simulink model "test_controller"  (R2020a)
settings: Solver=ode1  StartTime=0.0  StopTime=100  FixedStep=0.01  RelTol=1e-3
InitFcn:
  | Initialization;
values from neighbouring files (symbols this model uses):
  g_I = [0 0 9.8]'    [Disturbance_rotor_payload_ini.m]    (also in Initialization.m = [0 0 g]'; parameter_verification_1drone.m = [0 0 g]')
  invJ_B1 = inv(J)    [Disturbance_rotor_payload_ini.m]    (also in Initialization.m)
  J = [2 0.3 -0.5;0.3 1 0.2;-0.5 0.2 3]*10^-2    [Disturbance_rotor_payload_ini.m]    (also in Initialization.m)
  K_0 = 5    [Initialization.m]
  k_L = 0.15    [Initialization.m]
  K_omega = 1*eye(3)    [Disturbance_rotor_payload_ini.m]    (also in Initialization.m)
  k_p = 0.10    (= 0.1)    [Initialization.m]
  K_q = 100    [Disturbance_rotor_payload_ini.m]    (also in Initialization.m)
  K_R = 1*eye(3)    [Disturbance_rotor_payload_ini.m]    (also in Initialization.m)
  k_v = 7    [Disturbance_rotor_payload_ini.m]    (also in Initialization.m = 0.24)
  kappa = 0.9    [Initialization.m]
  Kr = 0.2    [Initialization.m]    (also in parameter_verification_1drone.m)
  L = 1    [Disturbance_rotor_payload_ini.m]    (also in Initialization.m = 0.98; parameter_verification_1drone.m = 0.98)
  Lambda = 0.4    [Initialization.m]    (also in parameter_verification_1drone.m)
  Lambda_initalB01 = angle2quat(initial_Euler(3),initial_Euler(2),initial_Euler(1))    [Disturbance_rotor_payload_ini.m]    (also in Initialization.m)
  lambda_p = 0.2    [Disturbance_rotor_payload_ini.m]    (also in Initialization.m)
  lambda_q = 0.3    [Disturbance_rotor_payload_ini.m]    (also in Initialization.m)
  Lambda_T = 0.5    [Initialization.m]
  m_p = 0.5    [Disturbance_rotor_payload_ini.m]    (also in Initialization.m; parameter_verification_1drone.m)
  m_q = 1.63    [Disturbance_rotor_payload_ini.m]    (also in Initialization.m)
  n_1 = [0 1 0]'    [Disturbance_rotor_payload_ini.m]    (also in Initialization.m)
  omega_b01 = [0.1 0.3 0]'    [Disturbance_rotor_payload_ini.m]    (also in Initialization.m)
  P_1 = [5 0 -6]'    [Disturbance_rotor_payload_ini.m]    (also in Initialization.m)
  U_initial = [y_dot_initial;v_q]    [Disturbance_rotor_payload_ini.m]    (also in Initialization.m)
  W_p = [-0.4 0.8 -0.3]'    [Disturbance_rotor_payload_ini.m]    (also in Initialization.m)
  W_q = [-1 2 -0.3]'    [Disturbance_rotor_payload_ini.m]    (also in Initialization.m)
  X_initial = [0 0 0]'    [Disturbance_rotor_payload_ini.m]    (also in Initialization.m)
  y_inital = [0.02 -0.02]'    [Disturbance_rotor_payload_ini.m]    (also in Initialization.m)
libraries: sharedtransform x2, dspinverses x2, dspmtrx3 x1, sharedutil x1
(part 1 of 2)
settings Model: Creator=arthus  LastModifiedBy=hs293go
settings DataIOCC: ReturnWorkspaceOutputs=off
settings DebuggingCC: ArithmeticOperatorsInVariantConditions=warning
settings SFSimCC: SimUseLocalCustomCode=off  CustomCodeUndefinedFunction=UseInterfaceOnly
settings RTWCC: RTWUseLocalCustomCode=off
settings CodeAppCC: StateflowObjectComments=on

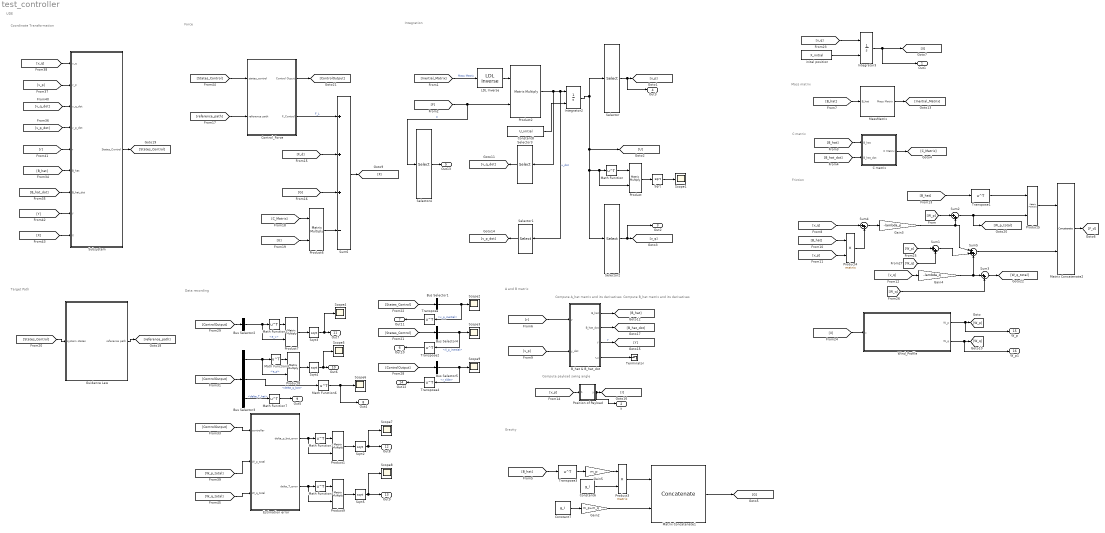
== system test_controller ==
  note: UDE
  note: Compute payload swing angle
  note: Integration
  note: Compute A_hat matrix and its derivatives
  note: Compute B_hat matrix and its derivatives
  note: Mass matrix
  note: A and B matrix
  note: Force
  note: C matrix
  note: Gravity
  note: Friction
  note: Data recording
  note: Coordinate Transformation
  note: Target Path
  B_hat & B_hat_dot : Subsystem
  Bus Selector1 : BusSelector  OutputSignals=v_p_inertial
  Bus Selector2 : BusSelector  OutputSignals=e_v
  Bus Selector3 : BusSelector  OutputSignals=e_p,delta_q_bot,delta_T_hat
  Bus Selector4 : BusSelector  OutputSignals=X_p_inertial
  Bus Selector5 : BusSelector  OutputSignals=r_tilde
  C matrix : Subsystem
  Constant6 : Constant  Value=g_I  VectorParams1D=off
  Constant7 : Constant  Value=g_I  VectorParams1D=off
  Constant8 : Constant  Value=U_initial  VectorParams1D=off
  Control_Force : Subsystem
  Estimation error : Subsystem
  Gain2 : Gain  Gain=m_p+m_q
  Gain3 : Gain  Gain=-lambda_p
  Gain4 : Gain  Gain=-lambda_q
  Gain5 : Gain  Gain=m_p
  "Guidance Law " : Subsystem
  Integrator2 : Integrator  InitialConditionSource=external  InitialCondition=U_initial
  Integrator3 : Integrator  InitialConditionSource=external
  LDL Inverse : dspinverses/LDL Inverse  errmode=Error
      settings: SourceProductBaseCode=DS
  MassMatrix : Subsystem
  Math Function{,1..4,6..7} (7 alike) : Math  Operator=transpose  SignedPower=on  SaturateOnIntegerOverflow=on
  Matrix Concatenate1 : Concatenate  Mode=Multidimensional array
  Matrix Concatenate2 : Concatenate  Mode=Multidimensional array
  Position of Payload : Subsystem
  Product{,1,3..9} (9 alike) : Product  Multiplication=Matrix(*)
  Product2 : Product  Multiplication=Matrix(*)  RndMeth=Zero
  Scope{1..9} (9 alike) : Scope
  Selector : Selector  InputPortWidth=5  IndexOptions=Index vector (dialog)  Indices=[1 2]  OutputSizes=1
  Selector1 : Selector  InputPortWidth=5  IndexOptions=Index vector (dialog)  Indices=[1 2]  OutputSizes=1
  Selector2 : Selector  InputPortWidth=5  IndexOptions=Index vector (dialog)  Indices=[3 4 5]  OutputSizes=1
  Selector3 : Selector  InputPortWidth=5  IndexOptions=Index vector (dialog)  Indices=[3 4 5]  OutputSizes=1
  Selector4 : Selector  InputPortWidth=5  IndexOptions=Index vector (dialog)  Indices=[3 4 5]  OutputSizes=1
  Sqrt{,2..5} (5 alike) : Sqrt  SaturateOnIntegerOverflow=on
  Subsystem : Subsystem
  Sum{1..4} (4 alike) : Sum  Inputs=|++
  Sum5 : Sum  Inputs=|+++
  Sum6 : Sum  Inputs=+++-
  Terminator : Terminator
  Transpose{,1..4} (5 alike) : Math  Operator=transpose  SignedPower=on  SaturateOnIntegerOverflow=on
  Wind_Profile : Subsystem
  inital position : Constant  Value=X_initial
  Out1 : Outport  SignalName=uav_pos
  y : Outport  Port=2  SignalName=pld_rel_pos
  Out2 : Outport  Port=3  SignalName=uav_vel
  Out3 : Outport  Port=4  SignalName=pld_rel_vel
  Out13 : Outport  Port=5  SignalName=act_force
  Out10 : Outport  Port=6  SignalName=pld_abs_pos
  Out11 : Outport  Port=7  SignalName=pld_abs_vel
  Out4 : Outport  Port=8  SignalName=proj_de
  Out5 : Outport  Port=9  SignalName=total_de
  Out6 : Outport  Port=10  SignalName=pos_err
  Out7 : Outport  Port=11  SignalName=vel_err
  Out8 : Outport  Port=12  SignalName=proj_de_est_err
  Out9 : Outport  Port=13  SignalName=total_de_est_err
  Out12 : Outport  Port=14  SignalName=pld_swing_est_err
  W_p : Outport  Port=15  SignalName=pld_dtb
  W_p1 : Outport  Port=16  SignalName=uav_dtb
  wires:
  ? -> ?
  Math Function7/1 -> Out5/1
  Bus Selector3/3 -> Math Function7/1  "<delta_T_hat>"
  Math Function6/1 -> Out4/1, Scope6/1
  Transpose4/1 -> Out12/1
  Bus Selector5/1 -> Transpose4/1, Scope9/1  "<r_tilde>"
  [ControlOutput] -> Bus Selector5/1
  Transpose2/1 -> Out10/1
  Transpose/1 -> Out11/1
  [W_q_total] -> Estimation error/3(W_q_total)
  Sum3/1 -> [W_q_total]
  [W_q] -> Sum3/2
  Bus Selector3/2 -> Math Function6/1  "<delta_q_bot>"
  Sqrt5/1 -> Out9/1, Scope8/1
  Estimation error/2(delta_T_error) -> Product9/2, Math Function4/1
  Math Function4/1 -> Product9/1
  Product9/1 -> Sqrt5/1
  Sqrt2/1 -> Out8/1, Scope7/1
  Estimation error/1(delta_p_bot_error) -> Product1/2, Math Function1/1
  Math Function1/1 -> Product1/1
  Product1/1 -> Sqrt2/1
  [W_p_total] -> Estimation error/2(W_p_total)
  [ControlOutput] -> Estimation error/1(controller)
  [States_Control] -> Bus Selector4/1
  Bus Selector4/1 -> Transpose2/1, Scope3/1  "<X_p_inertial>"
  Bus Selector1/1 -> Transpose/1, Scope2/1  "<v_p_inertial>"
  [States_Control] -> Bus Selector1/1
  [ControlOutput] -> Bus Selector3/1
  [ControlOutput] -> Bus Selector2/1
  Math Function3/1 -> Product8/1
  Bus Selector3/1 -> Product8/2, Math Function3/1  "<e_p>"
  Sqrt4/1 -> Out6/1, Scope5/1
  Product8/1 -> Sqrt4/1
  Bus Selector2/1 -> Product7/2, Math Function2/1  "<e_v>"
  Sqrt3/1 -> Out7/1, Scope4/1
  Product7/1 -> Sqrt3/1
  Math Function2/1 -> Product7/1
  Control_Force/1(Control Ouput) -> [ControlOutput]
  Control_Force/2(F_Control) -> Sum6/1  "F_L"
  [States_Control] -> "Guidance Law "/1(system states)
  "Guidance Law "/1(reference path) -> [reference_path]
  [reference_path] -> Control_Force/2(reference path)
  [X] -> Subsystem/9(X)
  [Y] -> Subsystem/8(Y)
  [r] -> Subsystem/5(r)
  [v_q_dot] -> Subsystem/3(v_q_dot)
  [v_q] -> Subsystem/1(v_q)
  [v_p] -> Subsystem/2(v_p)
  [v_p_dot] -> Subsystem/4(v_p_dot)
  [B_hat] -> Subsystem/6(B_hat)
  [B_hat_dot] -> Subsystem/7(B_hat_dot)
  Subsystem/1(States_Control) -> [States_Control]
  Selector1/1 -> [v_p_dot]
  Selector3/1 -> [v_q_dot]
  Selector/1 -> Out3/1, [v_p]
  [X] -> Wind_Profile/1(x)
  Wind_Profile/2(W_q) -> W_p1/1, [W_q]
  Sqrt/1 -> Scope1/1
  Product/1 -> Sqrt/1
  Math Function/1 -> Product/1
  [W_p] -> Sum1/1
  [W_q] -> Sum1/2
  [W_p] -> Sum2/1
  Wind_Profile/1(W_p) -> W_p/1, [W_p]
  B_hat & B_hat_dot/3(Y) -> [Y]  "Y"
  Gain3/1 -> Sum2/2, Sum5/1
  Sum2/1 -> [W_p_total], Product5/2
  Sum1/1 -> Sum5/2
  Gain4/1 -> Sum3/1, Sum5/3
  Integrator3/1 -> Out1/1, [X]
  B_hat & B_hat_dot/4(r_z) -> Terminator/1
  [States_Control] -> Control_Force/1(states_control)
  Constant8/1 -> Integrator2/2
  [v_q] -> Integrator3/1
  inital position/1 -> Integrator3/2
  Product6/1 -> Sum6/4
  [U] -> Product6/2
  [C_Matrix] -> Product6/1
  [G] -> Sum6/3
  [F_d] -> Sum6/2
  Sum6/1 -> [F]
  [v_p] -> Position of Payload/1(y_dot)
  Position of Payload/1(y) -> y/1, [r]
  Product5/1 -> Matrix Concatenate2/1
  Transpose1/1 -> Product5/1
  [B_hat] -> Transpose1/1
  [v_q] -> Gain4/1
  Product4/1 -> Sum4/2
  [v_p] -> Product4/2
  [B_hat] -> Product4/1
  [v_q] -> Sum4/1
  Sum4/1 -> Gain3/1
  Sum5/1 -> Matrix Concatenate2/2
  Matrix Concatenate2/1 -> [F_d]
  Matrix Concatenate1/1 -> [G]
  Gain2/1 -> Matrix Concatenate1/2
  Constant7/1 -> Gain2/1
  Product3/1 -> Matrix Concatenate1/1
  Transpose3/1 -> Gain5/1
  Constant6/1 -> Product3/2
  Gain5/1 -> Product3/1
  [B_hat] -> Transpose3/1
  [B_hat_dot] -> C matrix/2(B_hat_dot)
  [B_hat] -> C matrix/1(B_hat)
  C matrix/1(C Matrix) -> [C_Matrix]
  Selector2/1 -> Out2/1, [v_q]
  Integrator2/1 -> Selector/1, [U], Product/2, Math Function/1, Selector2/1
  Product2/1 -> Selector3/1, Selector1/1, Integrator2/1  "u_dot"
  [F] -> Selector4/1, Product2/2  "F"
  [Inertial_Matrix] -> LDL Inverse/1  "Mass Matrix"
  LDL Inverse/1 -> Product2/1
  [B_hat] -> MassMatrix/1(B_hat)
  [v_p] -> B_hat & B_hat_dot/2(y_dot)
  [r] -> B_hat & B_hat_dot/1(y)
  B_hat & B_hat_dot/1(B_hat) -> [B_hat]
  B_hat & B_hat_dot/2(B_hat_dot) -> [B_hat_dot]
  MassMatrix/1(Mass Matrix) -> [Inertial_Matrix]
  Selector4/1 -> Out13/1

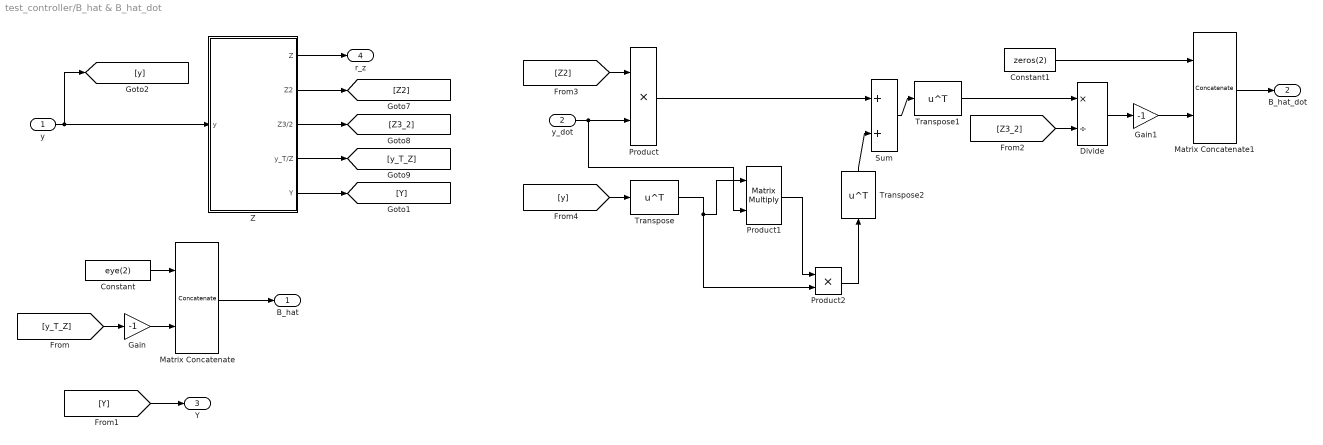
== system test_controller/B_hat & B_hat_dot ==
  y : Inport
  y_dot : Inport  Port=2
  Constant : Constant  Value=eye(2)
  Constant1 : Constant  Value=zeros(2)
  Divide : Product  Inputs=*/
  Gain : Gain  Gain=-1
  Gain1 : Gain  Gain=-1
  Matrix Concatenate : Concatenate  Mode=Multidimensional array
  Matrix Concatenate1 : Concatenate  Mode=Multidimensional array
  Product : Product  RndMeth=Zero
  Product1 : Product  Multiplication=Matrix(*)  RndMeth=Zero
  Product2 : Product  RndMeth=Zero
  Sum : Sum
  Transpose : Math  Operator=transpose  SignedPower=on  SaturateOnIntegerOverflow=on
  Transpose1 : Math  Operator=transpose  SignedPower=on  SaturateOnIntegerOverflow=on
  Transpose2 : Math  Operator=transpose  SignedPower=on  SaturateOnIntegerOverflow=on
  Z : Subsystem
  B_hat : Outport  VectorParamsAs1DForOutWhenUnconnected=off
  B_hat_dot : Outport  Port=2  VectorParamsAs1DForOutWhenUnconnected=off
  Y : Outport  Port=3  VectorParamsAs1DForOutWhenUnconnected=off
  r_z : Outport  Port=4  VectorParamsAs1DForOutWhenUnconnected=off
  wires:
  y_dot/1 -> Product/2, Product1/2
  y/1 -> Z/1(y), [y]
  Matrix Concatenate/1 -> B_hat/1
  Matrix Concatenate1/1 -> B_hat_dot/1
  Z/1(Z) -> r_z/1
  Z/2(Z2) -> [Z2]
  Z/3(Z3/2) -> [Z3_2]
  Z/4(y_T/Z) -> [y_T_Z]
  [y_T_Z] -> Gain/1
  Constant/1 -> Matrix Concatenate/1
  Gain/1 -> Matrix Concatenate/2
  Z/5(Y) -> [Y]
  [Y] -> Y/1
  Constant1/1 -> Matrix Concatenate1/1
  [Z3_2] -> Divide/2
  Sum/1 -> Transpose1/1
  [Z2] -> Product/1
  [y] -> Transpose/1
  Transpose/1 -> Product1/1, Product2/2
  Product1/1 -> Product2/1
  Divide/1 -> Gain1/1
  Gain1/1 -> Matrix Concatenate1/2
  Product2/1 -> Transpose2/1
  Product/1 -> Sum/1
  Transpose1/1 -> Divide/1
  Transpose2/1 -> Sum/2

== system test_controller/C matrix ==
  B_hat : Inport
  B_hat_dot : Inport  Port=2
  Constant : Constant  Value=[zeros(2,3);zeros(3)]  VectorParams1D=off
  Gain4 : Gain  Gain=m_p
  Gain5 : Gain  Gain=m_p
  Matrix Concatenate : Concatenate  Mode=Multidimensional array  ConcatenateDimension=2
  Matrix Concatenate1 : Concatenate  Mode=Multidimensional array
  Product1 : Product  Multiplication=Matrix(*)
  Transpose3 : Math  Operator=transpose  SignedPower=on  SaturateOnIntegerOverflow=on
  C Matrix : Outport  VectorParamsAs1DForOutWhenUnconnected=off
  wires:
  Matrix Concatenate/1 -> C Matrix/1
  Matrix Concatenate1/1 -> Matrix Concatenate/1
  Constant/1 -> Matrix Concatenate/2
  B_hat/1 -> Transpose3/1
  Transpose3/1 -> [B_hatT]
  Gain5/1 -> Matrix Concatenate1/1
  [B_hatT] -> Product1/1
  B_hat_dot/1 -> Gain4/1, Product1/2
  Product1/1 -> Gain5/1
  Gain4/1 -> Matrix Concatenate1/2

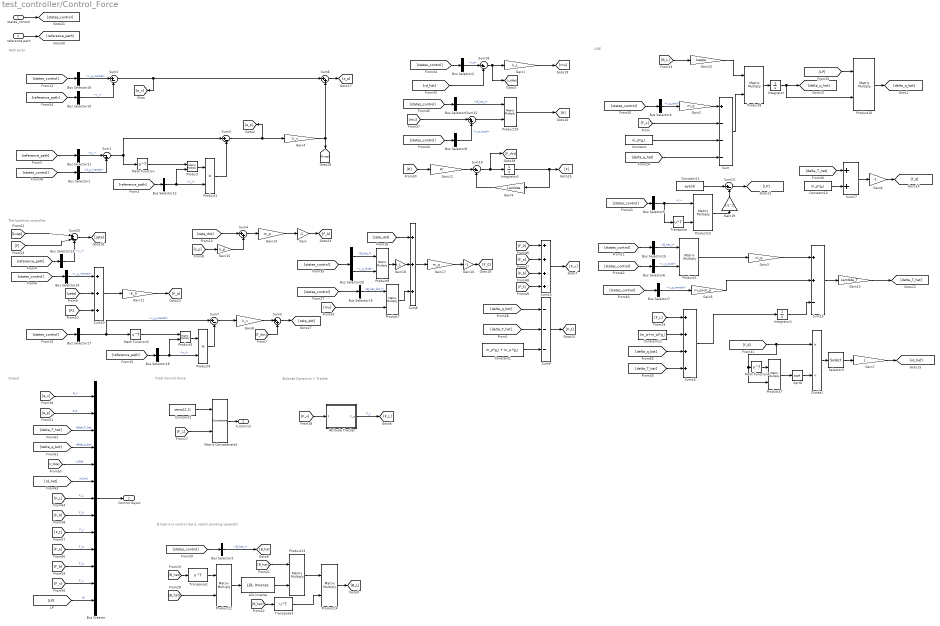
== system test_controller/Control_Force ==
  note: Output
  note: Path error
  note: The baseline controller
  note: Attitude Dynamics + Tracker
  note: B matrix in control law (L vector pointing upwards)
  note: UDE
  note: Total Control Force
  states_control : Inport
  reference path : Inport  Port=2
  Attitude Tracker : Subsystem
  Bus Creator : BusCreator  Inputs=13
  Bus Selector1 : BusSelector  OutputSignals=X_p_inertial
  Bus Selector10 : BusSelector  OutputSignals=v_i
  Bus Selector11 : BusSelector  OutputSignals=p_i
  Bus Selector12 : BusSelector  OutputSignals=n_i
  Bus Selector13 : BusSelector  OutputSignals=v_i
  Bus Selector{7,14,16..17} (4 alike) : BusSelector  OutputSignals=v_p_inertial
  Bus Selector15 : BusSelector  OutputSignals=B_hat_l
  Bus Selector18 : BusSelector  OutputSignals=n_i
  Bus Selector19 : BusSelector  OutputSignals=B_hat_dot_l
  Bus Selector2 : BusSelector  OutputSignals=r_q
  Bus Selector20 : BusSelector  OutputSignals=B_hat_l,v_q_local
  Bus Selector3 : BusSelector  OutputSignals=B_hat_l
  Bus Selector4 : BusSelector  OutputSignals=v_q_dot
  Bus Selector5 : BusSelector  OutputSignals=L
  Bus Selector6 : BusSelector  OutputSignals=v_q_local
  Bus Selector8 : BusSelector  OutputSignals=v_q_local
  Bus Selector9 : BusSelector  OutputSignals=B_hat_l
  Constant : Constant  Value=m_q*g_I
  Constant1 : Constant  Value=m_p*g_I + m_q *g_I
  Constant11 : Constant  Value=eye(3)
  Constant12 : Constant  Value=(m_p+m_q)*g_I
  Constant13 : Constant  Value=m_p*g_I
  Constant2 : Constant  Value=zeros(2,1)
  Divide1 : Product  Inputs=*/
  Gain : Gain  Gain=-1
  Gain1 : Gain  Gain=k_L
  Gain10 : Gain  Gain=kappa
  Gain11 : Gain  Gain=-K_0
  Gain12 : Gain  Gain=Kr
  Gain13 : Gain  Gain=Lambda_T
  Gain14 : Gain  Gain=m_p
  Gain15 : Gain  Gain=k_p
  Gain16 : Gain  Gain=-1
  Gain17 : Gain  Gain=m_q
  Gain18 : Gain  Gain=k_L
  Gain19 : Gain  Gain=1/L^2
  Gain2 : Gain  Gain=m_q
  Gain3 : Gain  Gain=m_q
  Gain4 : Gain  Gain=k_v
  Gain5 : Gain  Gain=m_q+m_p
  Gain6 : Gain  Gain=-1
  Gain7 : Gain  Gain=L
  Gain8 : Gain  Gain=k_v
  Gain9 : Gain  Gain=Lambda
  Integrator : Integrator
  Integrator1 : Integrator
  Integrator2 : Integrator
  LDL Inverse : dspinverses/LDL Inverse  errmode=Error
      settings: SourceProductBaseCode=DS
  Math Function : Math  Operator=transpose  SignedPower=on  SaturateOnIntegerOverflow=on
  Math Function3 : Math  Operator=transpose  SignedPower=on  SaturateOnIntegerOverflow=on
  Math Function4 : Math  Operator=transpose  SignedPower=on  SaturateOnIntegerOverflow=on
  Matrix Concatenate1 : Concatenate  Mode=Multidimensional array
  Product{,2..3,7..9,12..17,19} (13 alike) : Product  Multiplication=Matrix(*)
  Product1 : Product
  Product4 : Product
  Selector3 : Selector  InputPortWidth=3  IndexOptions=Index vector (dialog)  Indices=[1 2]  OutputSizes=1
  Sqrt6 : Sqrt  SaturateOnIntegerOverflow=on
  Sum : Sum  Inputs=+---
  Sum1 : Sum  Inputs=|-+
  Sum10 : Sum  Inputs=+++
  Sum{4..6,12} (4 alike) : Sum  Inputs=|++
  Sum{2..3,7,13,18..19} (6 alike) : Sum  Inputs=|+-
  Sum14 : Sum  Inputs=++++
  Sum15 : Sum  Inputs=++-
  Sum16 : Sum  Inputs=++++
  Sum17 : Sum
  Sum20 : Sum  Inputs=|++-
  Sum8 : Sum  Inputs=+++
  Sum9 : Sum  Inputs=---
  Transpose : Math  Operator=transpose  SignedPower=on  SaturateOnIntegerOverflow=on
  Transpose1 : Math  Operator=transpose  SignedPower=on  SaturateOnIntegerOverflow=on
  Transpose3 : Math  Operator=transpose  SignedPower=on  SaturateOnIntegerOverflow=on
  Control Ouput : Outport  VectorParamsAs1DForOutWhenUnconnected=off
  F_Control : Outport  Port=2  VectorParamsAs1DForOutWhenUnconnected=off
  wires:
  Constant2/1 -> Matrix Concatenate1/1
  Sum3/1 -> [e_p], Gain4/1
  Sum1/1 -> Sum3/1, Math Function/1
  Math Function/1 -> Product/1
  Product/1 -> Product1/1
  Product1/1 -> Sum3/2
  Bus Selector6/1 -> Product2/2  "<v_q_local>"
  Bus Selector7/1 -> Gain5/1  "<v_p_inertial>"
  Matrix Concatenate1/1 -> F_Control/1
  Attitude Tracker/1(F_q) -> [F_L]  "F_L"
  Sum2/1 -> [e_v], Sum6/1
  [F_L] -> Matrix Concatenate1/2
  [F_v] -> Attitude Tracker/1(F)
  Sum14/1 -> [F_v]
  [B_hat] -> Transpose1/1
  Transpose1/1 -> Product12/1
  [B_hat] -> Product12/2
  Product12/1 -> LDL Inverse/1
  LDL Inverse/1 -> Product13/2
  [B_hat] -> Product13/1
  Transpose3/1 -> Product14/2
  [B_hat] -> Transpose3/1
  Product13/1 -> Product14/1
  Product14/1 -> [B_L]
  [B_L] -> Gain10/1
  Gain10/1 -> Product8/1
  Integrator/1 -> Product16/2, [delta_q_hat]
  [delta_q_hat] -> Sum/4
  Constant/1 -> Sum/3
  [F_L] -> Sum/2
  Gain2/1 -> Sum/1
  Sum/1 -> Product8/2
  Product8/1 -> Integrator/1
  Constant11/1 -> Sum13/1
  Product15/1 -> Gain19/1
  Sum13/1 -> [LP]
  [LP] -> Product16/1
  Product16/1 -> [delta_q_bot]
  Bus Selector15/1 -> Product2/1  "<B_hat_l>"
  Product2/1 -> Gain3/1
  Gain3/1 -> Sum15/1
  Gain5/1 -> Sum15/2
  Sum15/1 -> Gain13/1
  Integrator1/1 -> Sum15/3
  [F_L] -> Sum16/1
  Constant12/1 -> Sum16/2
  [delta_q_bot] -> Sum16/3
  [delta_T_hat] -> Sum16/4
  [delta_T_hat] -> Sum17/1
  Constant13/1 -> Sum17/2
  Sum17/1 -> Gain6/1
  Gain6/1 -> [f_d]
  Selector3/1 -> Gain7/1
  Gain7/1 -> [rd_hat]
  Product17/1 -> Sqrt6/1
  [f_d] -> Product17/2, Math Function4/1, Divide1/1
  Divide1/1 -> Selector3/1
  Sqrt6/1 -> Divide1/2
  Math Function4/1 -> Product17/1
  Sum6/1 -> [s_p]
  Bus Selector16/1 -> Sum2/1  "<v_p_inertial>"
  Sum18/1 -> [r_tilde], Gain1/1
  Gain1/1 -> [mu]
  states_control/1 -> [states_control]
  [states_control] -> Bus Selector1/1
  Bus Selector1/1 -> Sum1/2  "<X_p_inertial>"
  [states_control] -> Bus Selector2/1
  Bus Selector2/1 -> Sum18/1  "<r_q>"
  [states_control] -> Bus Selector3/1
  Bus Selector3/1 -> [B_hat]  "<B_hat_l>"
  [states_control] -> Bus Selector4/1
  Bus Selector4/1 -> Gain2/1  "<v_q_dot>"
  [states_control] -> Bus Selector5/1
  Bus Selector5/1 -> Product15/1, Transpose/1  "<L>"
  [states_control] -> Bus Selector6/1
  [states_control] -> Bus Selector7/1
  [mu] -> Sum12/1
  Bus Selector8/1 -> Sum12/2  "<v_q_local>"
  [states_control] -> Bus Selector8/1
  Sum12/1 -> Product19/2
  Bus Selector9/1 -> Product19/1  "<B_hat_l>"
  [states_control] -> Bus Selector9/1
  Product19/1 -> [R]
  [F_0] -> Sum14/1
  [F_a] -> Sum14/2
  [F_b] -> Sum14/3
  [F_t] -> Sum14/4
  Integrator2/1 -> Gain9/1, [F]
  Sum19/1 -> [F_dot], Integrator2/1
  Gain9/1 -> Sum19/2
  [R] -> Gain12/1
  Gain12/1 -> Sum19/1
  Sum20/1 -> [zeta]
  Gain4/1 -> [kvep], Sum6/2
  [kvep] -> Sum20/1
  [F] -> Sum20/2
  reference path/1 -> [reference_path]
  [reference_path] -> Bus Selector10/1
  Bus Selector10/1 -> Sum2/2  "<v_i>"
  Bus Selector11/1 -> Sum1/1  "<p_i>"
  [reference_path] -> Bus Selector11/1
  [reference_path] -> Bus Selector12/1
  Bus Selector12/1 -> Product/2, Product1/2  "<n_i>"
  [reference_path] -> Bus Selector13/1
  Bus Selector13/1 -> Sum20/3  "<v_i>"
  Sum4/1 -> Gain14/1
  Gain16/1 -> [F_0]
  Gain11/1 -> [F_a]
  Sum9/1 -> [F_t]
  Sum10/1 -> Gain11/1
  Constant1/1 -> Sum9/3
  [states_control] -> Bus Selector14/1
  Bus Selector14/1 -> Sum10/1  "<v_p_inertial>"
  [zeta] -> Sum10/2
  [R] -> Sum10/3
  Sum16/1 -> Integrator1/1
  [delta_q_bot] -> Sum9/1
  [rd_hat] -> Sum18/2
  Gain13/1 -> [delta_T_hat]
  [states_control] -> Bus Selector15/1
  [delta_T_hat] -> Sum9/2
  [states_control] -> Bus Selector16/1
  Gain/1 -> [F_b]
  [F_dot] -> Sum5/2
  Sum5/1 -> [zeta_dot]
  [zeta_dot] -> Sum4/1
  Gain14/1 -> Gain/1
  Gain15/1 -> Sum4/2
  [s_p] -> Gain15/1
  Gain8/1 -> Sum5/1
  [states_control] -> Bus Selector17/1
  Bus Selector17/1 -> Sum7/1, Math Function3/1  "<v_p_inertial>"
  [reference_path] -> Bus Selector18/1
  Bus Selector18/1 -> Product3/2, Product4/2  "<n_i>"
  Product3/1 -> Product4/1
  Math Function3/1 -> Product3/1
  Product4/1 -> Sum7/2
  Sum7/1 -> Gain8/1
  Gain17/1 -> Gain16/1
  Sum8/1 -> Gain17/1
  [zeta_dot] -> Sum8/1
  Gain18/1 -> Sum8/2
  [states_control] -> Bus Selector19/1
  Bus Selector19/1 -> Product7/1  "<B_hat_dot_l>"
  Product7/1 -> Sum8/3
  [mu] -> Product7/2
  Product9/1 -> Gain18/1
  Bus Selector20/1 -> Product9/1  "<B_hat_l>"
  [states_control] -> Bus Selector20/1
  Bus Selector20/2 -> Product9/2  "<v_q_local>"
  Bus Creator/1 -> Control Ouput/1
  [e_v] -> Bus Creator/1  "e_v"
  [e_p] -> Bus Creator/2  "e_p"
  [delta_T_hat] -> Bus Creator/3  "delta_T_hat"
  [delta_q_bot] -> Bus Creator/4  "delta_q_bot"
  [r_tilde] -> Bus Creator/5  "r_tilde"
  [rd_hat] -> Bus Creator/6  "rd_hat"
  [F_L] -> Bus Creator/7  "F_L"
  [F_0] -> Bus Creator/8  "F_0"
  [F_t] -> Bus Creator/9  "F_t"
  [F_a] -> Bus Creator/10  "F_a"
  [F_b] -> Bus Creator/11  "F_b"
  [F_v] -> Bus Creator/12  "F_v"
  [LP] -> Bus Creator/13  "LP"
  Gain19/1 -> Sum13/2
  Transpose/1 -> Product15/2

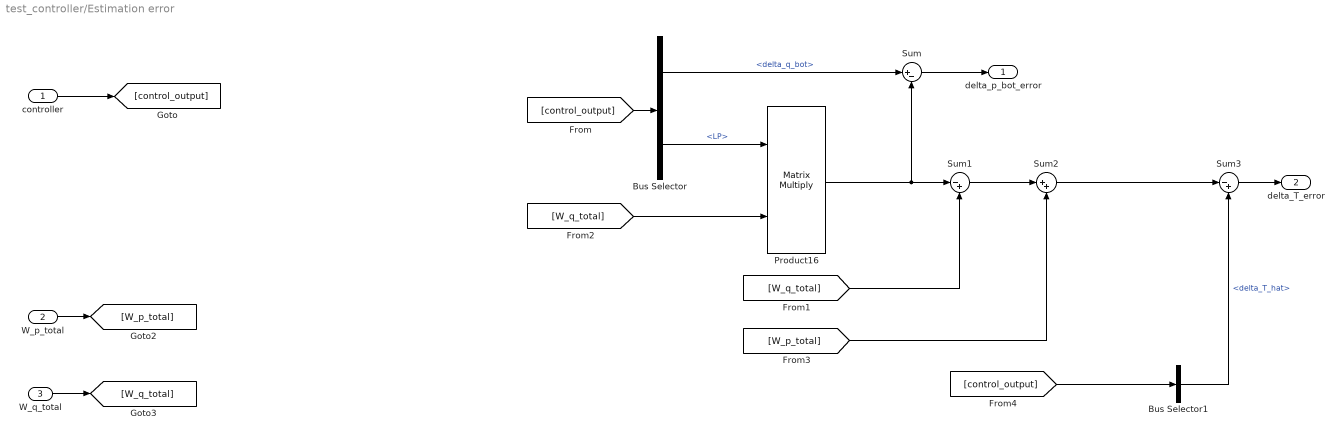
== system test_controller/Estimation error ==
  controller : Inport
  W_p_total : Inport  Port=2
  W_q_total : Inport  Port=3
  Bus Selector : BusSelector  OutputSignals=delta_q_bot,LP
  Bus Selector1 : BusSelector  OutputSignals=delta_T_hat
  Product16 : Product  Multiplication=Matrix(*)
  Sum : Sum  Inputs=|+-
  Sum1 : Sum  Inputs=|-+
  Sum2 : Sum  Inputs=|++
  Sum3 : Sum  Inputs=|-+
  delta_p_bot_error : Outport  VectorParamsAs1DForOutWhenUnconnected=off
  delta_T_error : Outport  Port=2  VectorParamsAs1DForOutWhenUnconnected=off
  wires:
  controller/1 -> [control_output]
  W_p_total/1 -> [W_p_total]
  W_q_total/1 -> [W_q_total]
  [control_output] -> Bus Selector/1
  Bus Selector/1 -> Sum/1  "<delta_q_bot>"
  Bus Selector/2 -> Product16/1  "<LP>"
  [W_q_total] -> Product16/2
  Product16/1 -> Sum1/1, Sum/2
  Sum/1 -> delta_p_bot_error/1
  Sum3/1 -> delta_T_error/1
  [W_q_total] -> Sum1/2
  Sum1/1 -> Sum2/1
  [W_p_total] -> Sum2/2
  Sum2/1 -> Sum3/1
  [control_output] -> Bus Selector1/1
  Bus Selector1/1 -> Sum3/2  "<delta_T_hat>"

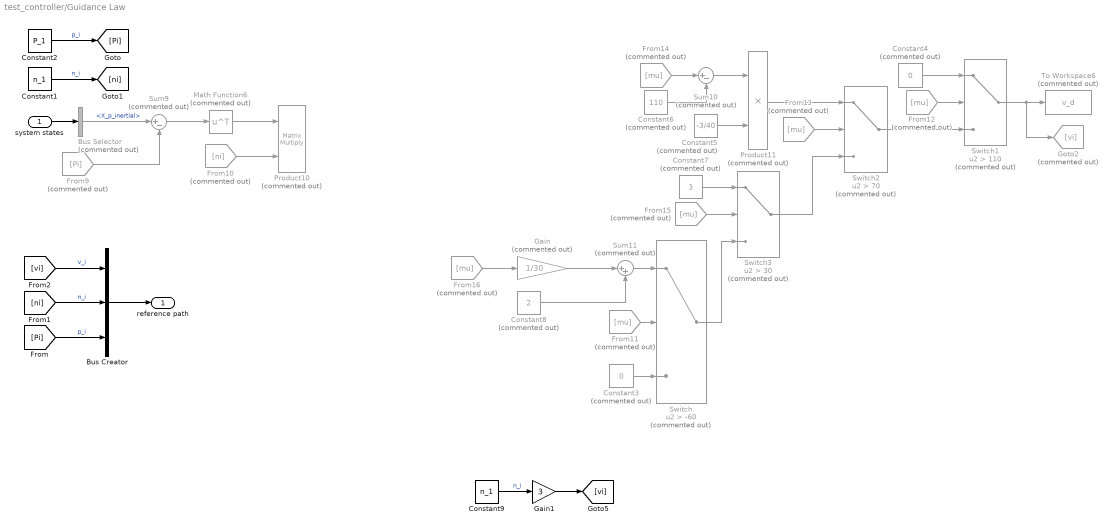
== system test_controller/Guidance Law  ==
  system states : Inport
  Bus Creator : BusCreator  Inputs=3
  Bus Selector : BusSelector  Commented=on  OutputSignals=X_p_inertial
  Constant1 : Constant  Value=n_1
  Constant2 : Constant  Value=P_1
  Constant3 : Constant  Commented=on  Value=0
  Constant4 : Constant  Commented=on  Value=0
  Constant5 : Constant  Commented=on  Value=-3/40
  Constant6 : Constant  Commented=on  Value=110
  Constant7 : Constant  Commented=on  Value=3
  Constant8 : Constant  Commented=on  Value=2
  Constant9 : Constant  Value=n_1
  From10 : From  Commented=on  GotoTag=ni
  From{11..16} (6 alike) : From  Commented=on  GotoTag=mu
  From9 : From  Commented=on  GotoTag=Pi
  Gain : Gain  Commented=on  Gain=1/30
  Gain1 : Gain  Gain=3
  Goto2 : Goto  Commented=on  GotoTag=vi
  Math Function6 : Math  Commented=on  Operator=transpose  SignedPower=on  SaturateOnIntegerOverflow=on
  Product10 : Product  Commented=on  Multiplication=Matrix(*)
  Product11 : Product  Commented=on
  Sum10 : Sum  Commented=on  Inputs=|+-
  Sum11 : Sum  Commented=on  Inputs=|++
  Sum9 : Sum  Commented=on  Inputs=|+-
  Switch : Switch  Commented=on  Criteria=u2 > Threshold  Threshold=-60
  Switch1 : Switch  Commented=on  Criteria=u2 > Threshold  Threshold=110
  Switch2 : Switch  Commented=on  Criteria=u2 > Threshold  Threshold=70
  Switch3 : Switch  Commented=on  Criteria=u2 > Threshold  Threshold=30
  To Workspace6 : ToWorkspace  Commented=on  VariableName=v_d  SaveFormat=Structure With Time  SampleTime=-1
  reference path : Outport  VectorParamsAs1DForOutWhenUnconnected=off
  wires:
  Sum11/1 -> Switch/1
  Math Function6/1 -> Product10/1
  From10/1 -> Product10/2
  Constant8/1 -> Sum11/2
  From9/1 -> Sum9/2
  Constant7/1 -> Switch3/1
  From13/1 -> Switch2/2
  Product11/1 -> Switch2/1
  Constant5/1 -> Product11/2
  From14/1 -> Sum10/1
  Switch2/1 -> Switch1/3
  Gain/1 -> Sum11/1
  Switch3/1 -> Switch2/3
  From16/1 -> Gain/1
  Constant4/1 -> Switch1/1
  Switch/1 -> Switch3/3
  Sum10/1 -> Product11/1
  Switch1/1 -> Goto2/1, To Workspace6/1
  Sum9/1 -> Math Function6/1
  From12/1 -> Switch1/2
  Constant6/1 -> Sum10/2
  From11/1 -> Switch/2
  From15/1 -> Switch3/2
  Bus Selector/1 -> Sum9/1  "<X_p_inertial>"
  Bus Creator/1 -> reference path/1
  Constant2/1 -> [Pi]  "p_i"
  system states/1 -> Bus Selector/1
  [Pi] -> Bus Creator/3  "p_i"
  Constant1/1 -> [ni]  "n_i"
  [ni] -> Bus Creator/2  "n_i"
  [vi] -> Bus Creator/1  "v_i"
  Constant3/1 -> Switch/3
  Constant9/1 -> Gain1/1  "n_i"
  Gain1/1 -> [vi]

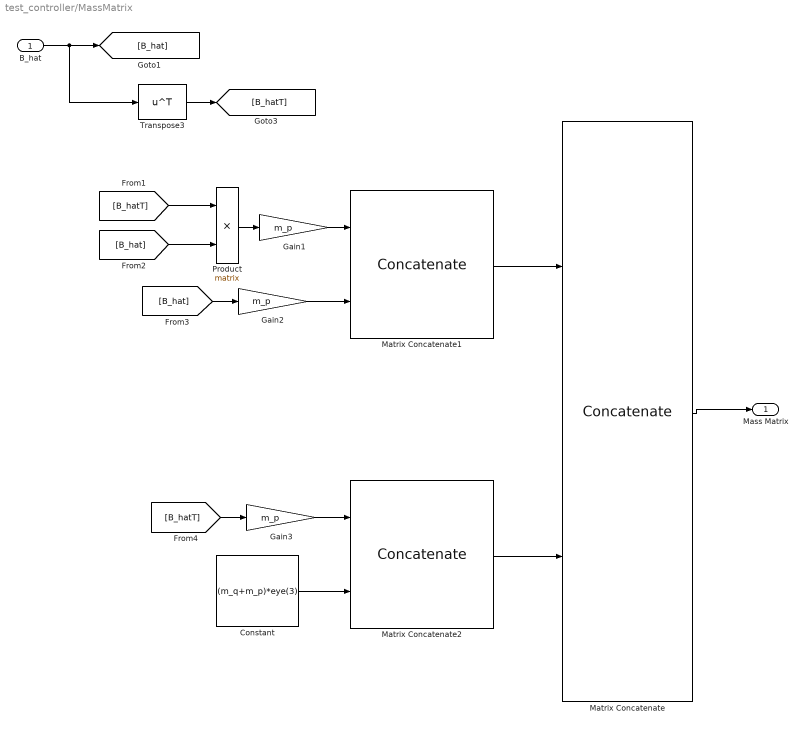
== system test_controller/MassMatrix ==
  B_hat : Inport
  Constant : Constant  Value=(m_q+m_p)*eye(3)
  Gain1 : Gain  Gain=m_p
  Gain2 : Gain  Gain=m_p
  Gain3 : Gain  Gain=m_p
  Matrix Concatenate : Concatenate  Mode=Multidimensional array  ConcatenateDimension=2
  Matrix Concatenate1 : Concatenate  Mode=Multidimensional array
  Matrix Concatenate2 : Concatenate  Mode=Multidimensional array
  Product : Product  Multiplication=Matrix(*)
  Transpose3 : Math  Operator=transpose  SignedPower=on  SaturateOnIntegerOverflow=on
  Mass Matrix : Outport  VectorParamsAs1DForOutWhenUnconnected=off
  wires:
  Matrix Concatenate/1 -> Mass Matrix/1
  Matrix Concatenate1/1 -> Matrix Concatenate/1
  Matrix Concatenate2/1 -> Matrix Concatenate/2
  B_hat/1 -> [B_hat], Transpose3/1
  Transpose3/1 -> [B_hatT]
  [B_hatT] -> Product/1
  [B_hat] -> Product/2
  Product/1 -> Gain1/1
  Gain1/1 -> Matrix Concatenate1/1
  Gain2/1 -> Matrix Concatenate1/2
  [B_hat] -> Gain2/1
  Constant/1 -> Matrix Concatenate2/2
  [B_hatT] -> Gain3/1
  Gain3/1 -> Matrix Concatenate2/1

== system test_controller/Position of Payload ==
  y_dot : Inport
  Integrator : Integrator  InitialConditionSource=external
  inital position : Constant  Value=y_inital  VectorParams1D=off
  y : Outport  VectorParamsAs1DForOutWhenUnconnected=off
  wires:
  Integrator/1 -> y/1
  y_dot/1 -> Integrator/1
  inital position/1 -> Integrator/2

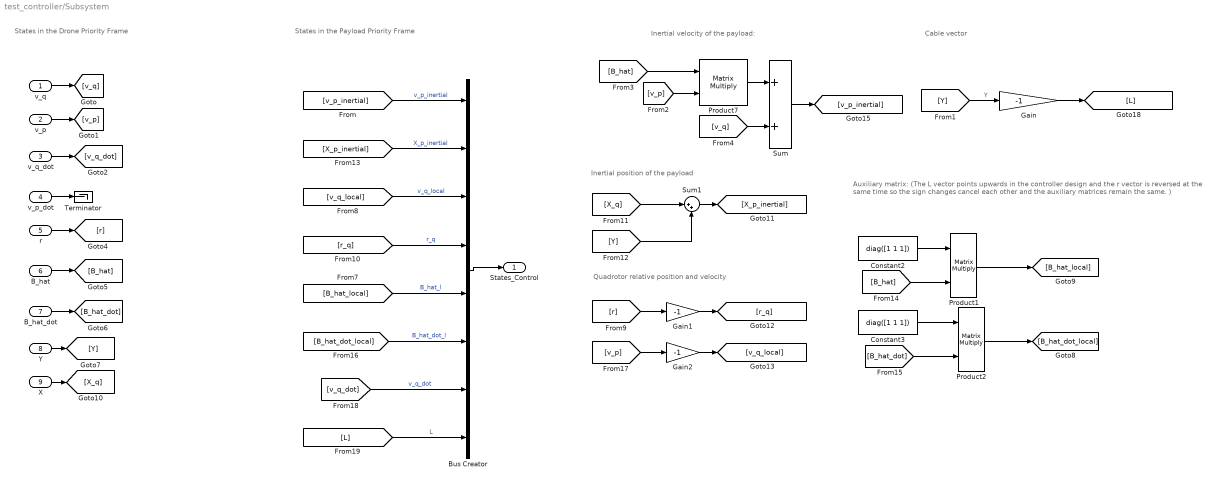
== system test_controller/Subsystem ==
  note: Quadrotor relative position and velocity
  note: Auxiliary matrix: (The L vector points upwards in the controller design and the r vector is reversed at the same time so
      | the sign changes cancel each other and the auxiliary matrices remain the same.  )
  note: Inertial position of the payload
  note: Cable vector
  note: Inertial velocity of the payload:
  note: States in the Drone Priority Frame
  note: States in the Payload Priority Frame
  v_q : Inport
  v_p : Inport  Port=2
  v_q_dot : Inport  Port=3
  v_p_dot : Inport  Port=4
  r : Inport  Port=5
  B_hat : Inport  Port=6
  B_hat_dot : Inport  Port=7
  Y : Inport  Port=8
  X : Inport  Port=9
  Bus Creator : BusCreator  Inputs=8
  Constant2 : Constant  Value=diag([1 1 1])
  Constant3 : Constant  Value=diag([1 1 1])
  Gain : Gain  Gain=-1
  Gain1 : Gain  Gain=-1
  Gain2 : Gain  Gain=-1
  Product1 : Product  Multiplication=Matrix(*)
  Product2 : Product  Multiplication=Matrix(*)
  Product7 : Product  Multiplication=Matrix(*)
  Sum : Sum
  Sum1 : Sum  Inputs=|++
  Terminator : Terminator
  States_Control : Outport  VectorParamsAs1DForOutWhenUnconnected=off
  wires:
  Bus Creator/1 -> States_Control/1
  Product7/1 -> Sum/1
  Sum/1 -> [v_p_inertial]
  [v_q] -> Sum/2
  [Y] -> Gain/1  "Y"
  Gain/1 -> [L]
  v_q/1 -> [v_q]
  v_p/1 -> [v_p]
  v_q_dot/1 -> [v_q_dot]
  v_p_dot/1 -> Terminator/1
  r/1 -> [r]
  B_hat/1 -> [B_hat]
  B_hat_dot/1 -> [B_hat_dot]
  Y/1 -> [Y]
  X/1 -> [X_q]
  [X_q] -> Sum1/1
  [Y] -> Sum1/2
  Sum1/1 -> [X_p_inertial]
  [r] -> Gain1/1
  Gain1/1 -> [r_q]
  [v_p_inertial] -> Bus Creator/1  "v_p_inertial"
  [X_p_inertial] -> Bus Creator/2  "X_p_inertial"
  [v_q_local] -> Bus Creator/3  "v_q_local"
  [r_q] -> Bus Creator/4  "r_q"
  [B_hat_local] -> Bus Creator/5  "B_hat_l"
  [B_hat_dot_local] -> Bus Creator/6  "B_hat_dot_l"
  [B_hat] -> Product1/2
  Product1/1 -> [B_hat_local]
  [B_hat_dot] -> Product2/2
  Product2/1 -> [B_hat_dot_local]
  [v_p] -> Gain2/1
  Gain2/1 -> [v_q_local]
  [v_q_dot] -> Bus Creator/7  "v_q_dot"
  [L] -> Bus Creator/8  "L"
  [v_p] -> Product7/2
  [B_hat] -> Product7/1
  Constant2/1 -> Product1/1
  Constant3/1 -> Product2/1

== system test_controller/Wind_Profile ==
  note: Constant wind profile is used
  x : Inport
  Constant1 : Constant  Value=W_p
  Constant2 : Constant  Value=W_q
  Terminator : Terminator
  W_p : Outport  VectorParamsAs1DForOutWhenUnconnected=off
  W_q : Outport  Port=2  VectorParamsAs1DForOutWhenUnconnected=off
  wires:
  x/1 -> Terminator/1
  Constant2/1 -> W_q/1
  Constant1/1 -> W_p/1

== system test_controller/B_hat & B_hat_dot/Z ==
  y : Inport
  Constant : Constant  Value=L^2  VectorParams1D=off
  Divide : Product  Inputs=*/
  Dot Product : DotProduct  InputSameDT=on  OutDataTypeStr=Inherit: Inherit via internal rule
  Dot Product1 : DotProduct  InputSameDT=on  OutDataTypeStr=Inherit: Inherit via internal rule
  Matrix Concatenate : Concatenate  ConcatenateDimension=2
  Sqrt : Sqrt  SaturateOnIntegerOverflow=on
  Sum : Sum  Inputs=|-+
  Transpose2 : Math  Operator=transpose  SignedPower=on  SaturateOnIntegerOverflow=on
  Z : Outport  VectorParamsAs1DForOutWhenUnconnected=off
  Z2 : Outport  Port=2  VectorParamsAs1DForOutWhenUnconnected=off
  Z3/2 : Outport  Port=3  VectorParamsAs1DForOutWhenUnconnected=off
  y_T/Z : Outport  Port=4  VectorParamsAs1DForOutWhenUnconnected=off
  Y : Outport  Port=5  VectorParamsAs1DForOutWhenUnconnected=off
  wires:
  y/1 -> Divide/1, Matrix Concatenate/1, Dot Product/2, Dot Product/1
  Constant/1 -> Sum/2
  Dot Product/1 -> Sum/1
  Sum/1 -> Sqrt/1, Z2/1, Dot Product1/2
  Sqrt/1 -> Dot Product1/1, Divide/2, Z/1, Matrix Concatenate/2
  Dot Product1/1 -> Z3/2/1
  Divide/1 -> Transpose2/1
  Transpose2/1 -> y_T/Z/1
  Matrix Concatenate/1 -> Y/1

== system test_controller/Control_Force/Attitude Tracker ==
  F : Inport
  Attitude Dynamics : Subsystem
  Attitude Tracker : Subsystem
  Atttitude Extraction : Subsystem
  Constant : Constant  Value=[0 0 1]'  VectorParams1D=off
  Divide : Product  Inputs=*/
  Dot Product : DotProduct  InputSameDT=on  OutDataTypeStr=Inherit: Inherit via internal rule
  Product : Product  Multiplication=Matrix(*)
  Product1 : Product
  Sqrt : Sqrt  SaturateOnIntegerOverflow=on
  Terminator : Terminator
  Terminator1 : Terminator
  F_q : Outport  VectorParamsAs1DForOutWhenUnconnected=off
  wires:
  F/1 -> Dot Product/2, Dot Product/1, Divide/1
  Constant/1 -> Product/2
  Product/1 -> Product1/2  "n_z"
  Product1/1 -> F_q/1
  Sqrt/1 -> Product1/1, Divide/2
  Dot Product/1 -> Sqrt/1
  Atttitude Extraction/1(R_d) -> Attitude Tracker/1(R_d)
  Atttitude Extraction/2(omega_d) -> Attitude Tracker/2(omega_d)
  Atttitude Extraction/3(omega_d_dot) -> Attitude Tracker/3(omega_d_dot)
  Divide/1 -> Atttitude Extraction/1(n_d)  "n1"
  Attitude Dynamics/4(omega_b) -> Attitude Tracker/5(omega)
  Attitude Dynamics/3(Euler) -> Terminator1/1  "Euler"
  Attitude Dynamics/2(RBI) -> Terminator/1
  Attitude Tracker/1(Torque_in_body_frame) -> Attitude Dynamics/1(MB)  "Mq_b"
  Attitude Dynamics/1(RIB) -> Attitude Tracker/4(R), Product/1  "IRB"

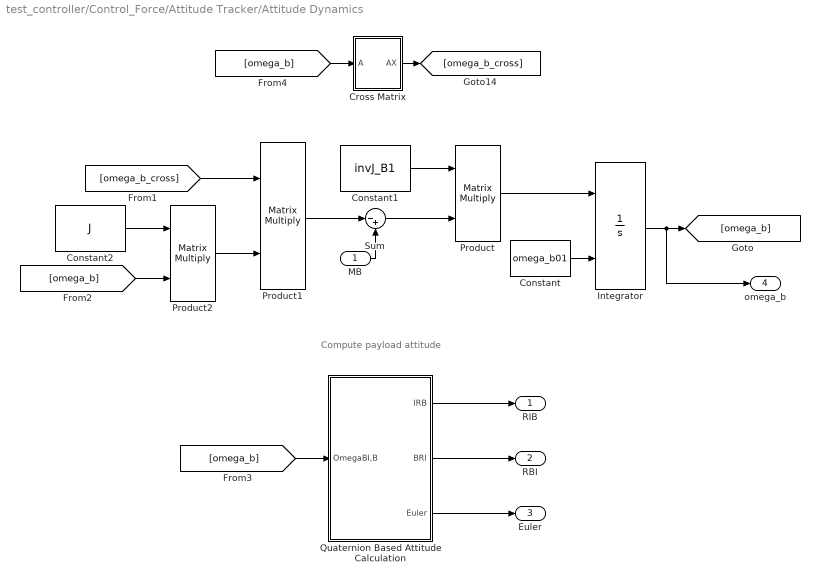
== system test_controller/Control_Force/Attitude Tracker/Attitude Dynamics ==
  note: Compute payload attitude
  MB : Inport
  Constant : Constant  Value=omega_b01  VectorParams1D=off
  Constant1 : Constant  Value=invJ_B1  VectorParams1D=off
  Constant2 : Constant  Value=J  VectorParams1D=off
  Cross Matrix : Subsystem
  Integrator : Integrator  InitialConditionSource=external
  Product : Product  Multiplication=Matrix(*)
  Product1 : Product  Multiplication=Matrix(*)
  Product2 : Product  Multiplication=Matrix(*)
  Quaternion Based Attitude Calculation : Subsystem
  Sum : Sum  Inputs=|-+
  RIB : Outport  VectorParamsAs1DForOutWhenUnconnected=off
  RBI : Outport  Port=2  VectorParamsAs1DForOutWhenUnconnected=off
  Euler : Outport  Port=3  VectorParamsAs1DForOutWhenUnconnected=off
  omega_b : Outport  Port=4  VectorParamsAs1DForOutWhenUnconnected=off
  wires:
  [omega_b] -> Cross Matrix/1(A)
  Cross Matrix/1(AX) -> [omega_b_cross]
  [omega_b] -> Quaternion Based Attitude Calculation/1(OmegaBI,B)
  Quaternion Based Attitude Calculation/1(IRB) -> RIB/1
  Quaternion Based Attitude Calculation/2(BRI) -> RBI/1
  Quaternion Based Attitude Calculation/3(Euler) -> Euler/1
  Integrator/1 -> omega_b/1, [omega_b]
  Constant/1 -> Integrator/2
  Product/1 -> Integrator/1
  Constant1/1 -> Product/1
  Sum/1 -> Product/2
  MB/1 -> Sum/2
  [omega_b_cross] -> Product1/1
  Product2/1 -> Product1/2
  Constant2/1 -> Product2/1
  [omega_b] -> Product2/2
  Product1/1 -> Sum/1

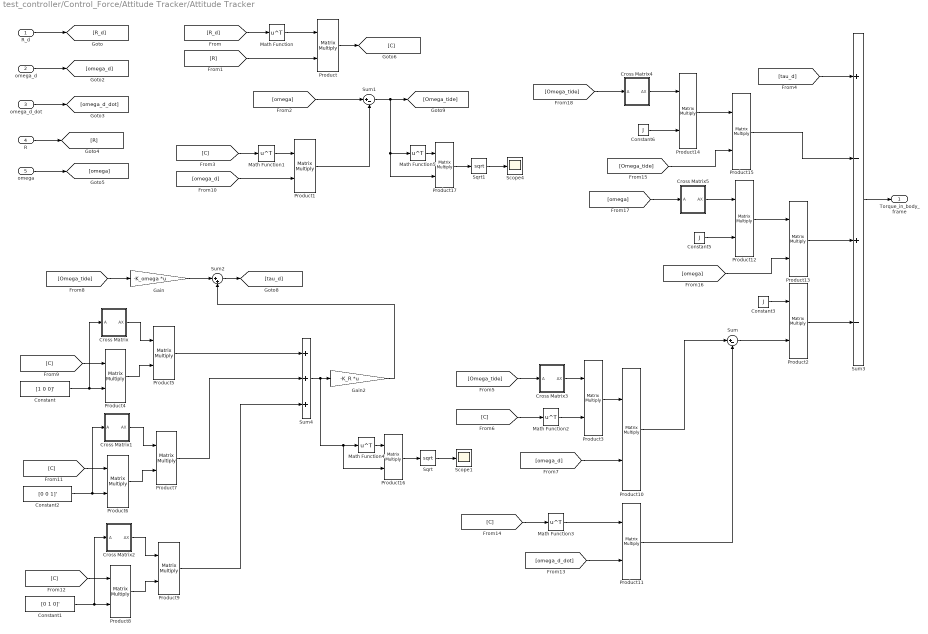
== system test_controller/Control_Force/Attitude Tracker/Attitude Tracker ==
  R_d : Inport
  omega_d : Inport  Port=2
  omega_d_dot : Inport  Port=3
  R : Inport  Port=4
  omega : Inport  Port=5
  Constant : Constant  Value=[1 0 0]'
  Constant1 : Constant  Value=[0 1 0]'
  Constant2 : Constant  Value=[0 0 1]'
  Constant3 : Constant  Value=J  VectorParams1D=off
  Constant5 : Constant  Value=J  VectorParams1D=off
  Constant6 : Constant  Value=J  VectorParams1D=off
  Cross Matrix : Subsystem
  Cross Matrix1 : Subsystem
  Cross Matrix2 : Subsystem
  Cross Matrix3 : Subsystem
  Cross Matrix4 : Subsystem
  Cross Matrix5 : Subsystem
  Gain : Gain  Gain=-K_omega  Multiplication=Matrix(K*u)
  Gain2 : Gain  Gain=-K_R  Multiplication=Matrix(K*u)
  Math Function{,1..5} (6 alike) : Math  Operator=transpose  SignedPower=on  SaturateOnIntegerOverflow=on
  Product{,1..17} (18 alike) : Product  Multiplication=Matrix(*)
  Scope1 : Scope
  Scope4 : Scope
  Sqrt : Sqrt  SaturateOnIntegerOverflow=on
  Sqrt1 : Sqrt  SaturateOnIntegerOverflow=on
  Sum : Sum  Inputs=|+-
  Sum1 : Sum  Inputs=|+-
  Sum2 : Sum  Inputs=|++
  Sum3 : Sum  Inputs=+-+-
  Sum4 : Sum  Inputs=+++
  Torque_in_body_frame : Outport  VectorParamsAs1DForOutWhenUnconnected=off
  wires:
  R_d/1 -> [R_d]
  omega_d/1 -> [omega_d]
  omega_d_dot/1 -> [omega_d_dot]
  [R_d] -> Math Function/1
  Math Function/1 -> Product/1
  R/1 -> [R]
  omega/1 -> [omega]
  [R] -> Product/2
  Product/1 -> [C]
  [C] -> Math Function1/1
  Math Function1/1 -> Product1/1
  [omega] -> Sum1/1
  Product1/1 -> Sum1/2
  [omega_d] -> Product1/2
  Sum2/1 -> [tau_d]
  Gain/1 -> Sum2/1
  [Omega_tide] -> Gain/1
  [tau_d] -> Sum3/1
  [C] -> Product4/1
  Constant/1 -> Cross Matrix/1(A), Product4/2
  Cross Matrix/1(AX) -> Product5/1
  Product4/1 -> Product5/2
  [C] -> Product6/1
  Constant2/1 -> Cross Matrix1/1(A), Product6/2
  Cross Matrix1/1(AX) -> Product7/1
  Product6/1 -> Product7/2
  Product7/1 -> Sum4/2
  [C] -> Product8/1
  Constant1/1 -> Cross Matrix2/1(A), Product8/2
  Cross Matrix2/1(AX) -> Product9/1
  Product8/1 -> Product9/2
  Product9/1 -> Sum4/3
  Product5/1 -> Sum4/1
  Gain2/1 -> Sum2/2
  Sum3/1 -> Torque_in_body_frame/1
  Constant3/1 -> Product2/1
  Sum/1 -> Product2/2
  [Omega_tide] -> Cross Matrix3/1(A)
  [C] -> Math Function2/1
  Cross Matrix3/1(AX) -> Product3/1
  Math Function2/1 -> Product3/2
  Product3/1 -> Product10/1
  [omega_d] -> Product10/2
  Product10/1 -> Sum/1
  [C] -> Math Function3/1
  Math Function3/1 -> Product11/1
  [omega_d_dot] -> Product11/2
  Product11/1 -> Sum/2
  Product2/1 -> Sum3/4
  Product13/1 -> Sum3/3
  Product12/1 -> Product13/1
  [omega] -> Product13/2
  [omega] -> Cross Matrix5/1(A)
  Cross Matrix5/1(AX) -> Product12/1
  Constant5/1 -> Product12/2
  Product14/1 -> Product15/1
  [Omega_tide] -> Product15/2
  [Omega_tide] -> Cross Matrix4/1(A)
  Cross Matrix4/1(AX) -> Product14/1
  Constant6/1 -> Product14/2
  Product15/1 -> Sum3/2
  Sum4/1 -> Product16/2, Math Function4/1, Gain2/1
  Math Function4/1 -> Product16/1
  Product16/1 -> Sqrt/1
  Sqrt/1 -> Scope1/1
  Sum1/1 -> Math Function5/1, Product17/2, [Omega_tide]
  Math Function5/1 -> Product17/1
  Product17/1 -> Sqrt1/1
  Sqrt1/1 -> Scope4/1

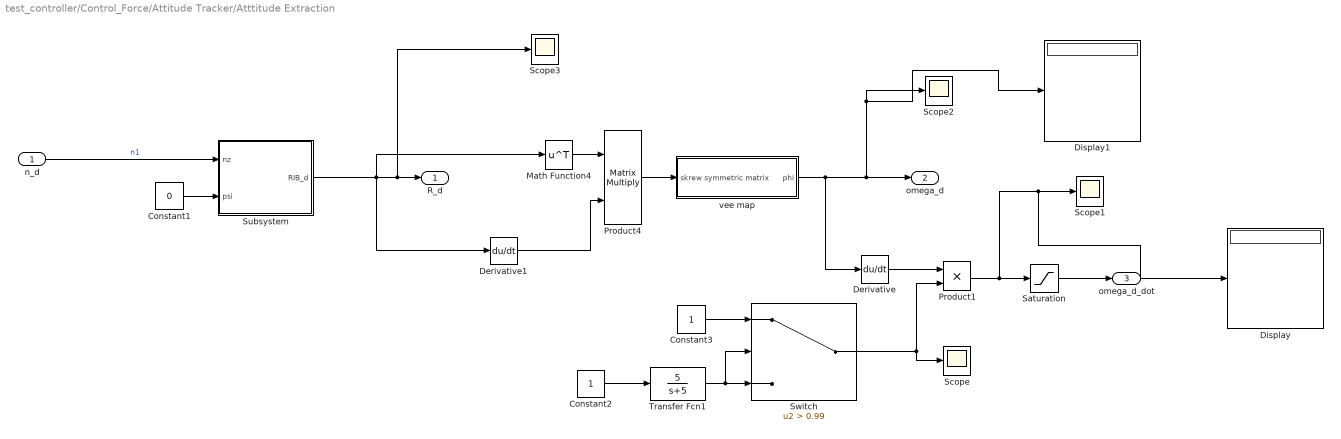
== system test_controller/Control_Force/Attitude Tracker/Atttitude Extraction ==
  n_d : Inport
  Constant1 : Constant  Value=0
  Constant2 : Constant
  Constant3 : Constant
  Derivative : Derivative
  Derivative1 : Derivative
  Display : Display
  Display1 : Display
  Math Function4 : Math  Operator=transpose  SignedPower=on  SaturateOnIntegerOverflow=on
  Product1 : Product
  Product4 : Product  Multiplication=Matrix(*)
  Saturation : Saturate  UpperLimit=10  LowerLimit=-10
  Scope{,1..3} (4 alike) : Scope
  Subsystem : Subsystem
  Switch : Switch  Criteria=u2 > Threshold  Threshold=0.99  ZeroCross=off
  Transfer Fcn1 : TransferFcn  Numerator=[5]  Denominator=[1 5]
  vee map : Subsystem
  R_d : Outport  VectorParamsAs1DForOutWhenUnconnected=off
  omega_d : Outport  Port=2  VectorParamsAs1DForOutWhenUnconnected=off
  omega_d_dot : Outport  Port=3  VectorParamsAs1DForOutWhenUnconnected=off
  wires:
  Math Function4/1 -> Product4/1
  Derivative1/1 -> Product4/2
  Product4/1 -> vee map/1(skrew symmetric matrix)
  vee map/1(phi) -> Derivative/1, Display1/1, Scope2/1, omega_d/1
  n_d/1 -> Subsystem/1(nz)  "n1"
  Constant1/1 -> Subsystem/2(psi)
  Subsystem/1(RIB_d) -> Derivative1/1, Math Function4/1, Scope3/1, R_d/1
  Constant2/1 -> Transfer Fcn1/1
  Derivative/1 -> Product1/1
  Product1/1 -> Display/1, Scope1/1, Saturation/1
  Switch/1 -> Scope/1, Product1/2
  Constant3/1 -> Switch/1
  Transfer Fcn1/1 -> Switch/2, Switch/3
  Saturation/1 -> omega_d_dot/1

== system test_controller/Control_Force/Attitude Tracker/Attitude Dynamics/Cross Matrix ==
  A : Inport
  Constant1 : Constant  Value=0  VectorParams1D=off
  Constant2 : Constant  Value=0  VectorParams1D=off
  Constant3 : Constant  Value=0  VectorParams1D=off
  Demux2 : Demux  Outputs=3
  Gain : Gain  Gain=-1
  Gain1 : Gain  Gain=-1
  Gain2 : Gain  Gain=-1
  Matrix Concatenate : Concatenate  NumInputs=3  Mode=Multidimensional array  ConcatenateDimension=2
  Matrix Concatenate1 : Concatenate  NumInputs=3  Mode=Multidimensional array
  Matrix Concatenate2 : Concatenate  NumInputs=3  Mode=Multidimensional array
  Matrix Concatenate3 : Concatenate  NumInputs=3  Mode=Multidimensional array
  AX : Outport  VectorParamsAs1DForOutWhenUnconnected=off
  wires:
  A/1 -> Demux2/1
  Demux2/1 -> Gain1/1, Matrix Concatenate2/3  "r1"
  Demux2/2 -> Gain2/1, Matrix Concatenate3/1  "r2"
  Matrix Concatenate/1 -> AX/1
  Demux2/3 -> Gain/1, Matrix Concatenate1/2  "r3"
  Matrix Concatenate1/1 -> Matrix Concatenate/1
  Matrix Concatenate2/1 -> Matrix Concatenate/2
  Constant2/1 -> Matrix Concatenate2/2
  Gain/1 -> Matrix Concatenate2/1
  Matrix Concatenate3/1 -> Matrix Concatenate/3
  Gain1/1 -> Matrix Concatenate3/2
  Constant3/1 -> Matrix Concatenate3/3
  Constant1/1 -> Matrix Concatenate1/1
  Gain2/1 -> Matrix Concatenate1/3

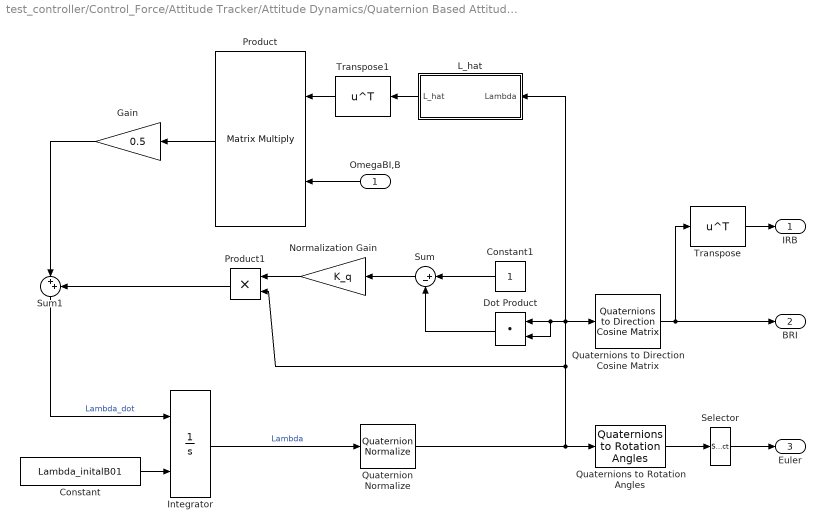
== system test_controller/Control_Force/Attitude Tracker/Attitude Dynamics/Quaternion Based Attitude Calculation ==
  OmegaBI,B : Inport
  Constant : Constant  Value=Lambda_initalB01
  Constant1 : Constant
  Dot Product : DotProduct  OutDataTypeStr=Inherit: Inherit via internal rule
  Gain : Gain  Gain=0.5
  Integrator : Integrator  InitialConditionSource=external
  L_hat : Subsystem
  Normalization Gain : Gain  Gain=K_q
  Product : Product  Multiplication=Matrix(*)  RndMeth=Zero
  Product1 : Product  RndMeth=Zero
  Quaternion Normalize : sharedutil/Quaternion Normalize  aMode=aMode
      settings: SourceProductBaseCode=AE,PW,MT,VE,VP
  Quaternions to Direction Cosine Matrix : sharedtransform/Quaternions to  Direction Cosine Matrix  aMode=aMode
      settings: SourceProductBaseCode=AE,PW,MT,VE,VP
  Quaternions to Rotation Angles : sharedtransform/Quaternions to Rotation Angles  rotationOrder=ZYX  aMode=aMode
      settings: SourceProductBaseCode=AE,PW,MT,VE,VP
  Selector : Selector  InputPortWidth=3  IndexOptions=Index vector (dialog)  Indices=[3 2 1]  OutputSizes=1
  Sum : Sum  Inputs=|+-  InputSameDT=on  SaturateOnIntegerOverflow=on  OutDataTypeStr=Inherit: Same as first input
  Sum1 : Sum  Inputs=|++
  Transpose : Math  Operator=transpose  SignedPower=on  SaturateOnIntegerOverflow=on
  Transpose1 : Math  Operator=transpose  SignedPower=on  SaturateOnIntegerOverflow=on
  IRB : Outport  VectorParamsAs1DForOutWhenUnconnected=off
  BRI : Outport  Port=2  VectorParamsAs1DForOutWhenUnconnected=off
  Euler : Outport  Port=3  VectorParamsAs1DForOutWhenUnconnected=off
  wires:
  Constant/1 -> Integrator/2
  Quaternions to Rotation Angles/1 -> Selector/1
  Selector/1 -> Euler/1
  Integrator/1 -> Quaternion Normalize/1  "Lambda"
  Sum1/1 -> Integrator/1  "Lambda_dot"
  Quaternions to Direction Cosine Matrix/1 -> BRI/1, Transpose/1
  Transpose/1 -> IRB/1
  Dot Product/1 -> Sum/2
  Constant1/1 -> Sum/1
  L_hat/1(L_hat) -> Transpose1/1
  Transpose1/1 -> Product/1
  OmegaBI,B/1 -> Product/2
  Sum/1 -> Normalization Gain/1
  Product/1 -> Gain/1
  Gain/1 -> Sum1/1
  Normalization Gain/1 -> Product1/1
  Product1/1 -> Sum1/2
  Quaternion Normalize/1 -> Quaternions to Rotation Angles/1, Quaternions to Direction Cosine Matrix/1, Dot Product/1, Dot Product/2, L_hat/1(Lambda), Product1/2

== system test_controller/Control_Force/Attitude Tracker/Attitude Tracker/Cross Matrix ==
  A : Inport
  Constant1 : Constant  Value=0  VectorParams1D=off
  Constant2 : Constant  Value=0  VectorParams1D=off
  Constant3 : Constant  Value=0  VectorParams1D=off
  Demux2 : Demux  Outputs=3
  Gain : Gain  Gain=-1
  Gain1 : Gain  Gain=-1
  Gain2 : Gain  Gain=-1
  Matrix Concatenate : Concatenate  NumInputs=3  Mode=Multidimensional array  ConcatenateDimension=2
  Matrix Concatenate1 : Concatenate  NumInputs=3  Mode=Multidimensional array
  Matrix Concatenate2 : Concatenate  NumInputs=3  Mode=Multidimensional array
  Matrix Concatenate3 : Concatenate  NumInputs=3  Mode=Multidimensional array
  AX : Outport  VectorParamsAs1DForOutWhenUnconnected=off
  wires:
  A/1 -> Demux2/1
  Demux2/1 -> Gain1/1, Matrix Concatenate2/3  "r1"
  Demux2/2 -> Gain2/1, Matrix Concatenate3/1  "r2"
  Matrix Concatenate/1 -> AX/1
  Demux2/3 -> Gain/1, Matrix Concatenate1/2  "r3"
  Matrix Concatenate1/1 -> Matrix Concatenate/1
  Matrix Concatenate2/1 -> Matrix Concatenate/2
  Constant2/1 -> Matrix Concatenate2/2
  Gain/1 -> Matrix Concatenate2/1
  Matrix Concatenate3/1 -> Matrix Concatenate/3
  Gain1/1 -> Matrix Concatenate3/2
  Constant3/1 -> Matrix Concatenate3/3
  Constant1/1 -> Matrix Concatenate1/1
  Gain2/1 -> Matrix Concatenate1/3

== system test_controller/Control_Force/Attitude Tracker/Attitude Tracker/Cross Matrix1 ==
  A : Inport
  Constant1 : Constant  Value=0  VectorParams1D=off
  Constant2 : Constant  Value=0  VectorParams1D=off
  Constant3 : Constant  Value=0  VectorParams1D=off
  Demux2 : Demux  Outputs=3
  Gain : Gain  Gain=-1
  Gain1 : Gain  Gain=-1
  Gain2 : Gain  Gain=-1
  Matrix Concatenate : Concatenate  NumInputs=3  Mode=Multidimensional array  ConcatenateDimension=2
  Matrix Concatenate1 : Concatenate  NumInputs=3  Mode=Multidimensional array
  Matrix Concatenate2 : Concatenate  NumInputs=3  Mode=Multidimensional array
  Matrix Concatenate3 : Concatenate  NumInputs=3  Mode=Multidimensional array
  AX : Outport  VectorParamsAs1DForOutWhenUnconnected=off
  wires:
  A/1 -> Demux2/1
  Demux2/1 -> Gain1/1, Matrix Concatenate2/3  "r1"
  Demux2/2 -> Gain2/1, Matrix Concatenate3/1  "r2"
  Matrix Concatenate/1 -> AX/1
  Demux2/3 -> Gain/1, Matrix Concatenate1/2  "r3"
  Matrix Concatenate1/1 -> Matrix Concatenate/1
  Matrix Concatenate2/1 -> Matrix Concatenate/2
  Constant2/1 -> Matrix Concatenate2/2
  Gain/1 -> Matrix Concatenate2/1
  Matrix Concatenate3/1 -> Matrix Concatenate/3
  Gain1/1 -> Matrix Concatenate3/2
  Constant3/1 -> Matrix Concatenate3/3
  Constant1/1 -> Matrix Concatenate1/1
  Gain2/1 -> Matrix Concatenate1/3

== system test_controller/Control_Force/Attitude Tracker/Attitude Tracker/Cross Matrix2 ==
  A : Inport
  Constant1 : Constant  Value=0  VectorParams1D=off
  Constant2 : Constant  Value=0  VectorParams1D=off
  Constant3 : Constant  Value=0  VectorParams1D=off
  Demux2 : Demux  Outputs=3
  Gain : Gain  Gain=-1
  Gain1 : Gain  Gain=-1
  Gain2 : Gain  Gain=-1
  Matrix Concatenate : Concatenate  NumInputs=3  Mode=Multidimensional array  ConcatenateDimension=2
  Matrix Concatenate1 : Concatenate  NumInputs=3  Mode=Multidimensional array
  Matrix Concatenate2 : Concatenate  NumInputs=3  Mode=Multidimensional array
  Matrix Concatenate3 : Concatenate  NumInputs=3  Mode=Multidimensional array
  AX : Outport  VectorParamsAs1DForOutWhenUnconnected=off
  wires:
  A/1 -> Demux2/1
  Demux2/1 -> Gain1/1, Matrix Concatenate2/3  "r1"
  Demux2/2 -> Gain2/1, Matrix Concatenate3/1  "r2"
  Matrix Concatenate/1 -> AX/1
  Demux2/3 -> Gain/1, Matrix Concatenate1/2  "r3"
  Matrix Concatenate1/1 -> Matrix Concatenate/1
  Matrix Concatenate2/1 -> Matrix Concatenate/2
  Constant2/1 -> Matrix Concatenate2/2
  Gain/1 -> Matrix Concatenate2/1
  Matrix Concatenate3/1 -> Matrix Concatenate/3
  Gain1/1 -> Matrix Concatenate3/2
  Constant3/1 -> Matrix Concatenate3/3
  Constant1/1 -> Matrix Concatenate1/1
  Gain2/1 -> Matrix Concatenate1/3

== system test_controller/Control_Force/Attitude Tracker/Attitude Tracker/Cross Matrix3 ==
  A : Inport
  Constant1 : Constant  Value=0  VectorParams1D=off
  Constant2 : Constant  Value=0  VectorParams1D=off
  Constant3 : Constant  Value=0  VectorParams1D=off
  Demux2 : Demux  Outputs=3
  Gain : Gain  Gain=-1
  Gain1 : Gain  Gain=-1
  Gain2 : Gain  Gain=-1
  Matrix Concatenate : Concatenate  NumInputs=3  Mode=Multidimensional array  ConcatenateDimension=2
  Matrix Concatenate1 : Concatenate  NumInputs=3  Mode=Multidimensional array
  Matrix Concatenate2 : Concatenate  NumInputs=3  Mode=Multidimensional array
  Matrix Concatenate3 : Concatenate  NumInputs=3  Mode=Multidimensional array
  AX : Outport  VectorParamsAs1DForOutWhenUnconnected=off
  wires:
  A/1 -> Demux2/1
  Demux2/1 -> Gain1/1, Matrix Concatenate2/3  "r1"
  Demux2/2 -> Gain2/1, Matrix Concatenate3/1  "r2"
  Matrix Concatenate/1 -> AX/1
  Demux2/3 -> Gain/1, Matrix Concatenate1/2  "r3"
  Matrix Concatenate1/1 -> Matrix Concatenate/1
  Matrix Concatenate2/1 -> Matrix Concatenate/2
  Constant2/1 -> Matrix Concatenate2/2
  Gain/1 -> Matrix Concatenate2/1
  Matrix Concatenate3/1 -> Matrix Concatenate/3
  Gain1/1 -> Matrix Concatenate3/2
  Constant3/1 -> Matrix Concatenate3/3
  Constant1/1 -> Matrix Concatenate1/1
  Gain2/1 -> Matrix Concatenate1/3

== system test_controller/Control_Force/Attitude Tracker/Attitude Tracker/Cross Matrix4 ==
  A : Inport
  Constant1 : Constant  Value=0  VectorParams1D=off
  Constant2 : Constant  Value=0  VectorParams1D=off
  Constant3 : Constant  Value=0  VectorParams1D=off
  Demux2 : Demux  Outputs=3
  Gain : Gain  Gain=-1
  Gain1 : Gain  Gain=-1
  Gain2 : Gain  Gain=-1
  Matrix Concatenate : Concatenate  NumInputs=3  Mode=Multidimensional array  ConcatenateDimension=2
  Matrix Concatenate1 : Concatenate  NumInputs=3  Mode=Multidimensional array
  Matrix Concatenate2 : Concatenate  NumInputs=3  Mode=Multidimensional array
  Matrix Concatenate3 : Concatenate  NumInputs=3  Mode=Multidimensional array
  AX : Outport  VectorParamsAs1DForOutWhenUnconnected=off
  wires:
  A/1 -> Demux2/1
  Demux2/1 -> Gain1/1, Matrix Concatenate2/3  "r1"
  Demux2/2 -> Gain2/1, Matrix Concatenate3/1  "r2"
  Matrix Concatenate/1 -> AX/1
  Demux2/3 -> Gain/1, Matrix Concatenate1/2  "r3"
  Matrix Concatenate1/1 -> Matrix Concatenate/1
  Matrix Concatenate2/1 -> Matrix Concatenate/2
  Constant2/1 -> Matrix Concatenate2/2
  Gain/1 -> Matrix Concatenate2/1
  Matrix Concatenate3/1 -> Matrix Concatenate/3
  Gain1/1 -> Matrix Concatenate3/2
  Constant3/1 -> Matrix Concatenate3/3
  Constant1/1 -> Matrix Concatenate1/1
  Gain2/1 -> Matrix Concatenate1/3

== system test_controller/Control_Force/Attitude Tracker/Attitude Tracker/Cross Matrix5 ==
  A : Inport
  Constant1 : Constant  Value=0  VectorParams1D=off
  Constant2 : Constant  Value=0  VectorParams1D=off
  Constant3 : Constant  Value=0  VectorParams1D=off
  Demux2 : Demux  Outputs=3
  Gain : Gain  Gain=-1
  Gain1 : Gain  Gain=-1
  Gain2 : Gain  Gain=-1
  Matrix Concatenate : Concatenate  NumInputs=3  Mode=Multidimensional array  ConcatenateDimension=2
  Matrix Concatenate1 : Concatenate  NumInputs=3  Mode=Multidimensional array
  Matrix Concatenate2 : Concatenate  NumInputs=3  Mode=Multidimensional array
  Matrix Concatenate3 : Concatenate  NumInputs=3  Mode=Multidimensional array
  AX : Outport  VectorParamsAs1DForOutWhenUnconnected=off
  wires:
  A/1 -> Demux2/1
  Demux2/1 -> Gain1/1, Matrix Concatenate2/3  "r1"
  Demux2/2 -> Gain2/1, Matrix Concatenate3/1  "r2"
  Matrix Concatenate/1 -> AX/1
  Demux2/3 -> Gain/1, Matrix Concatenate1/2  "r3"
  Matrix Concatenate1/1 -> Matrix Concatenate/1
  Matrix Concatenate2/1 -> Matrix Concatenate/2
  Constant2/1 -> Matrix Concatenate2/2
  Gain/1 -> Matrix Concatenate2/1
  Matrix Concatenate3/1 -> Matrix Concatenate/3
  Gain1/1 -> Matrix Concatenate3/2
  Constant3/1 -> Matrix Concatenate3/3
  Constant1/1 -> Matrix Concatenate1/1
  Gain2/1 -> Matrix Concatenate1/3
